simulink model "OrbitSimV1_export"  (R2021b)
settings: Solver=FixedStepAuto  StartTime=0.0  StopTime=1000  FixedStep=.01  RelTol=1e-3
model workspace (MAT data in the model file):
  orbit_altitude = 450000
  r_earth = 6378100
  vel_init = 7640
libraries: matrix_library x5, vrlib x4
settings Model: Creator=Ian Lee  LastModifiedBy=Ian Lee

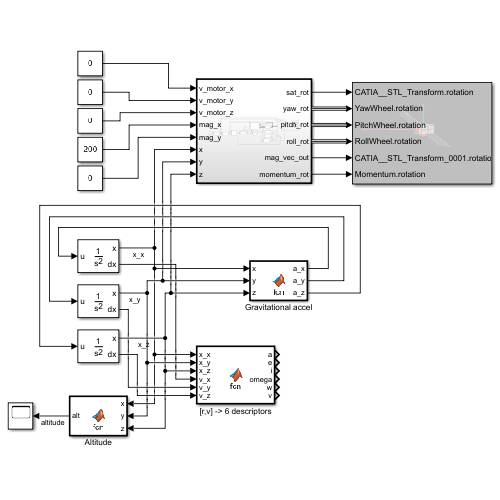
[thumbnail: Simulink's stored preview of the top-level diagram]
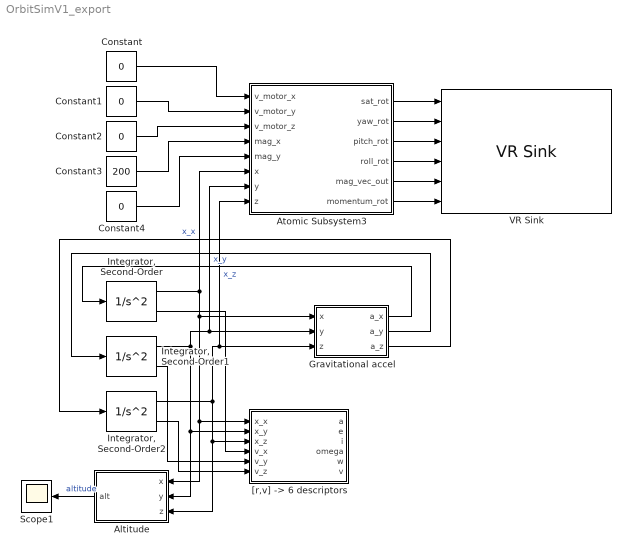
== system OrbitSimV1_export ==
  Altitude : MATLAB Function  TreatAsAtomicUnit=on
  Atomic Subsystem3 : Subsystem  TreatAsAtomicUnit=on
  Constant{,1..2,4} (4 alike) : Constant  Value=0
  Constant3 : Constant  Value=200
  Gravitational accel : MATLAB Function  TreatAsAtomicUnit=on
  "Integrator, Second-Order" : SecondOrderIntegrator  ICX=0  ICDXDT=5500
  "Integrator, Second-Order1" : SecondOrderIntegrator  ICX=r_earth + orbit_altitude  ICDXDT=0
  "Integrator, Second-Order2" : SecondOrderIntegrator  ICDXDT=5300
  Scope1 : Scope
  VR Sink : vrlib/VR Sink  InstantiateOnLoad=on  SampleTime=.02  ViewEnable=on  RemoteChange=off  RemoteView=off  FieldsWritten=CATIA__STL_Transform.rotation.4.1.1.double#YawWheel.rotation.4.1.1.double#PitchWheel.rotation.4.1.1.double#RollWheel.rotation.4.1.1.double#CATIA__STL_Transform_0001.rotation.4.1.1.double#Momentum.rotation.4.1.1.double  WorldFileName=SatVR.x3d  AutoView=off  VideoDimensions=[]  AllowVariableSize=off
  "[r,v] -> 6 descriptors" : MATLAB Function  TreatAsAtomicUnit=on
  wires:
  Gravitational accel/2(a_y) -> "Integrator, Second-Order1"/1
  Gravitational accel/1(a_x) -> "Integrator, Second-Order"/1
  Altitude/1(alt) -> Scope1/1  "altitude"
  "Integrator, Second-Order1"/1 -> "[r,v] -> 6 descriptors"/2(x_y), Altitude/2(y), Atomic Subsystem3/7(y), Gravitational accel/2(y)  "x_y"
  Gravitational accel/3(a_z) -> "Integrator, Second-Order2"/1
  "Integrator, Second-Order2"/1 -> "[r,v] -> 6 descriptors"/3(x_z), Altitude/3(z), Atomic Subsystem3/8(z), Gravitational accel/3(z)  "x_z"
  "Integrator, Second-Order"/1 -> Atomic Subsystem3/6(x), "[r,v] -> 6 descriptors"/1(x_x), Altitude/1(x), Gravitational accel/1(x)  "x_x"
  "Integrator, Second-Order"/2 -> "[r,v] -> 6 descriptors"/4(v_x)
  "Integrator, Second-Order1"/2 -> "[r,v] -> 6 descriptors"/5(v_y)
  "Integrator, Second-Order2"/2 -> "[r,v] -> 6 descriptors"/6(v_z)
  Atomic Subsystem3/1(sat_rot) -> VR Sink/1
  Atomic Subsystem3/2(yaw_rot) -> VR Sink/2
  Atomic Subsystem3/3(pitch_rot) -> VR Sink/3
  Atomic Subsystem3/4(roll_rot) -> VR Sink/4
  Atomic Subsystem3/5(mag_vec_out) -> VR Sink/5
  Atomic Subsystem3/6(momentum_rot) -> VR Sink/6
  Constant4/1 -> Atomic Subsystem3/5(mag_y)
  Constant3/1 -> Atomic Subsystem3/4(mag_x)
  Constant2/1 -> Atomic Subsystem3/3(v_motor_z)
  Constant1/1 -> Atomic Subsystem3/2(v_motor_y)
  Constant/1 -> Atomic Subsystem3/1(v_motor_x)

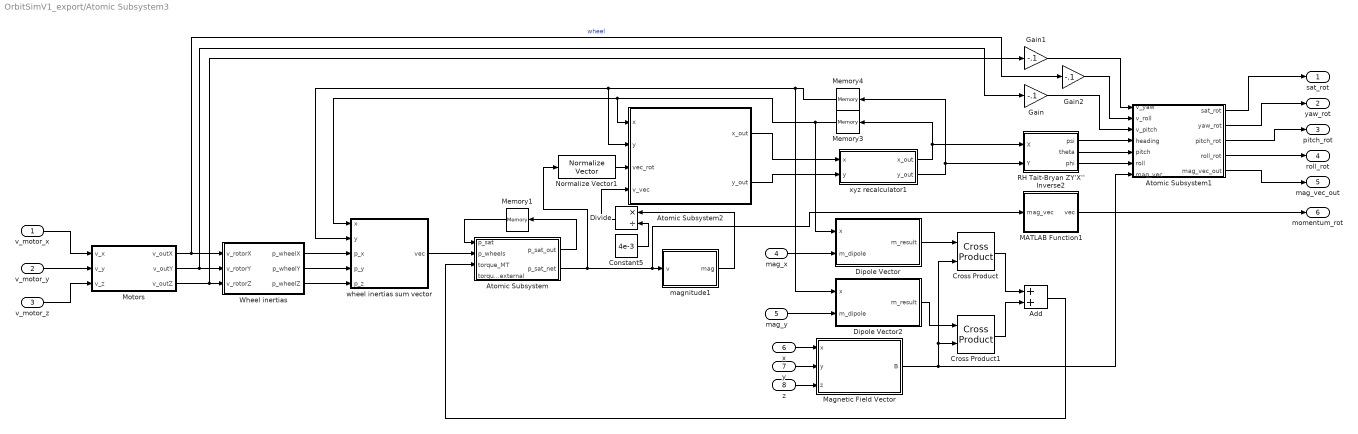
== system OrbitSimV1_export/Atomic Subsystem3 ==
  v_motor_x : Inport
  v_motor_y : Inport  Port=2
  v_motor_z : Inport  Port=3
  mag_x : Inport  Port=4
  mag_y : Inport  Port=5
  x : Inport  Port=6
  y : Inport  Port=7
  z : Inport  Port=8
  Add : Sum
  Atomic Subsystem : Subsystem  TreatAsAtomicUnit=on
  Atomic Subsystem1 : Subsystem  TreatAsAtomicUnit=on
  Atomic Subsystem2 : Subsystem  TreatAsAtomicUnit=on
      mask Display: image('C:\Users\benml\Downloads\imageMas.png'); % Use "Edit Image" on toolstrip to change.
  Constant5 : Constant  Value=4e-3
  Cross Product : matrix_library/Cross Product
      settings: SourceProductBaseCode=SL
  Cross Product1 : matrix_library/Cross Product
      settings: SourceProductBaseCode=SL
  Dipole Vector : MATLAB Function  TreatAsAtomicUnit=on
  Dipole Vector2 : MATLAB Function  TreatAsAtomicUnit=on
  Divide : Product  Inputs=*/
  Gain : Gain  Gain=-.1
  Gain1 : Gain  Gain=-.1
  Gain2 : Gain  Gain=-.1
  MATLAB Function1 : MATLAB Function  TreatAsAtomicUnit=on
  Magnetic Field Vector : MATLAB Function  TreatAsAtomicUnit=on
  Memory1 : Memory
  Memory3 : Memory  InitialCondition=[1,0,0]
  Memory4 : Memory  InitialCondition=[0,1,0]
  Motors : Subsystem  TreatAsAtomicUnit=on
  Normalize Vector1 : vrlib/Utilities/Normalize Vector  maxzero=0
  RH Tait-Bryan ZY'X'' Inverse2 : MATLAB Function  TreatAsAtomicUnit=on
  Wheel inertias : Subsystem  TreatAsAtomicUnit=on
  magnitude1 : MATLAB Function  TreatAsAtomicUnit=on
  wheel inertias sum vector : Subsystem  TreatAsAtomicUnit=on
  xyz recalculator1 : Subsystem  TreatAsAtomicUnit=on
  sat_rot : Outport
  yaw_rot : Outport  Port=2
  pitch_rot : Outport  Port=3
  roll_rot : Outport  Port=4
  mag_vec_out : Outport  Port=5
  momentum_rot : Outport  Port=6
  wires:
  wheel inertias sum vector/1(" vec") -> Atomic Subsystem/2(p_wheels)
  Atomic Subsystem/2(p_sat_net) -> MATLAB Function1/1(mag_vec), magnitude1/1(v), Normalize Vector1/1
  Normalize Vector1/1 -> Atomic Subsystem2/3(vec_rot)
  Memory1/1 -> Atomic Subsystem/1(p_sat)
  Atomic Subsystem/1(p_sat_out) -> Memory1/1
  Cross Product1/1 -> Add/2
  Add/1 -> Atomic Subsystem/3(torque_MT)
  Constant5/1 -> Divide/2
  Divide/1 -> Atomic Subsystem2/4(v_vec)
  xyz recalculator1/1(x_out) -> RH Tait-Bryan ZY'X'' Inverse2/1(X), Memory3/1
  RH Tait-Bryan ZY'X'' Inverse2/2(theta) -> Atomic Subsystem1/5(pitch)
  RH Tait-Bryan ZY'X'' Inverse2/1(psi) -> Atomic Subsystem1/4(heading)
  Atomic Subsystem2/1(x_out) -> xyz recalculator1/1(x)
  Cross Product/1 -> Add/1
  Gain/1 -> Atomic Subsystem1/3(v_pitch)
  MATLAB Function1/1(vec) -> momentum_rot/1
  Atomic Subsystem2/2(y_out) -> xyz recalculator1/2(y)
  Magnetic Field Vector/1(B) -> Cross Product/2, Cross Product1/2, Atomic Subsystem1/7(mag_vec)
  Gain2/1 -> Atomic Subsystem1/2(v_roll)
  Atomic Subsystem1/2(yaw_rot) -> yaw_rot/1
  Wheel inertias/3(p_wheelZ) -> wheel inertias sum vector/5(p_z)
  Atomic Subsystem1/3(pitch_rot) -> pitch_rot/1
  Motors/1(v_outX) -> Gain2/1, Wheel inertias/1(v_rotorX)  "wheel"
  xyz recalculator1/2(y_out) -> RH Tait-Bryan ZY'X'' Inverse2/2(Y), Memory4/1
  RH Tait-Bryan ZY'X'' Inverse2/3(phi) -> Atomic Subsystem1/6(roll)
  Motors/3(v_outZ) -> Gain1/1, Wheel inertias/3(v_rotorZ)
  Motors/2(v_outY) -> Gain/1, Wheel inertias/2(v_rotorY)
  Wheel inertias/2(p_wheelY) -> wheel inertias sum vector/4(p_y)
  Atomic Subsystem1/1(sat_rot) -> sat_rot/1
  Gain1/1 -> Atomic Subsystem1/1(v_yaw)
  Dipole Vector/1(m_result) -> Cross Product/1
  Memory3/1 -> Dipole Vector/1(x), wheel inertias sum vector/1(x), Atomic Subsystem2/1(x)
  Dipole Vector2/1(m_result) -> Cross Product1/1
  Atomic Subsystem1/5(mag_vec_out) -> mag_vec_out/1
  magnitude1/1(mag) -> Divide/1
  Memory4/1 -> Atomic Subsystem2/2(y), wheel inertias sum vector/2(y), Dipole Vector2/1(x)
  Wheel inertias/1(p_wheelX) -> wheel inertias sum vector/3(p_x)
  Atomic Subsystem1/4(roll_rot) -> roll_rot/1
  z/1 -> Magnetic Field Vector/3(z)
  y/1 -> Magnetic Field Vector/2(y)
  x/1 -> Magnetic Field Vector/1(x)
  v_motor_y/1 -> Motors/2(v_y)
  v_motor_x/1 -> Motors/1(v_x)
  v_motor_z/1 -> Motors/3(v_z)
  mag_x/1 -> Dipole Vector/2(m_dipole)
  mag_y/1 -> Dipole Vector2/2(m_dipole)

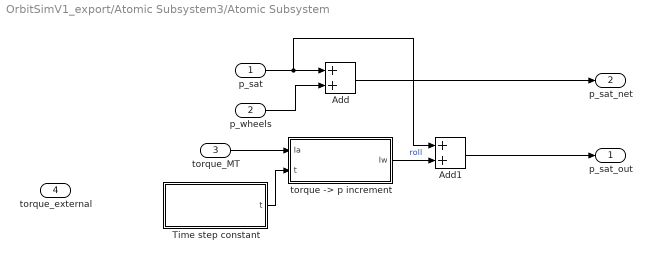
== system OrbitSimV1_export/Atomic Subsystem3/Atomic Subsystem ==
  p_sat : Inport
  p_wheels : Inport  Port=2
  torque_MT : Inport  Port=3
  torque_external : Inport  Port=4
  Add : Sum
  Add1 : Sum
  Time step constant : Subsystem  TreatAsAtomicUnit=on
  "torque -> p increment" : Subsystem  TreatAsAtomicUnit=on
  p_sat_out : Outport
  p_sat_net : Outport  Port=2
  wires:
  Time step constant/1(t) -> "torque -> p increment"/2(t)
  torque_MT/1 -> "torque -> p increment"/1(Ia)
  p_sat/1 -> Add1/1, Add/1
  p_wheels/1 -> Add/2
  Add/1 -> p_sat_net/1
  "torque -> p increment"/1(Iw) -> Add1/2  "roll"
  Add1/1 -> p_sat_out/1

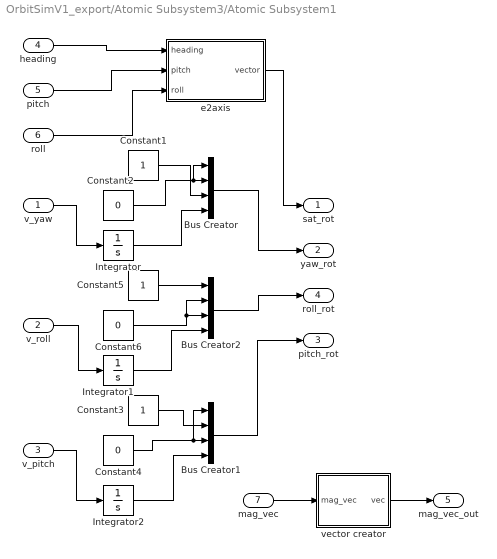
== system OrbitSimV1_export/Atomic Subsystem3/Atomic Subsystem1 ==
  v_yaw : Inport
  v_roll : Inport  Port=2
  v_pitch : Inport  Port=3
  heading : Inport  Port=4
  pitch : Inport  Port=5
  roll : Inport  Port=6
  mag_vec : Inport  Port=7
  Bus Creator : BusCreator  Inputs=4
  Bus Creator1 : BusCreator  Inputs=4
  Bus Creator2 : BusCreator  Inputs=4
  Constant1 : Constant
  Constant2 : Constant  Value=0
  Constant3 : Constant
  Constant4 : Constant  Value=0
  Constant5 : Constant
  Constant6 : Constant  Value=0
  Integrator : Integrator
  Integrator1 : Integrator
  Integrator2 : Integrator
  e2axis : MATLAB Function  TreatAsAtomicUnit=on
  vector creator : MATLAB Function  TreatAsAtomicUnit=on
  sat_rot : Outport
  yaw_rot : Outport  Port=2
  pitch_rot : Outport  Port=3
  roll_rot : Outport  Port=4
  mag_vec_out : Outport  Port=5
  wires:
  Constant6/1 -> Bus Creator2/2, Bus Creator2/3
  Constant5/1 -> Bus Creator2/1
  Constant1/1 -> Bus Creator/3
  Constant3/1 -> Bus Creator1/2
  Constant2/1 -> Bus Creator/1, Bus Creator/2
  Constant4/1 -> Bus Creator1/1, Bus Creator1/3
  heading/1 -> e2axis/1(heading)
  pitch/1 -> e2axis/2(pitch)
  roll/1 -> e2axis/3(roll)
  e2axis/1(vector) -> sat_rot/1
  v_yaw/1 -> Integrator/1
  v_roll/1 -> Integrator1/1
  v_pitch/1 -> Integrator2/1
  Bus Creator/1 -> yaw_rot/1
  Bus Creator2/1 -> roll_rot/1
  Bus Creator1/1 -> pitch_rot/1
  Integrator/1 -> Bus Creator/4
  Integrator1/1 -> Bus Creator2/4
  Integrator2/1 -> Bus Creator1/4
  mag_vec/1 -> vector creator/1(mag_vec)
  vector creator/1(vec) -> mag_vec_out/1

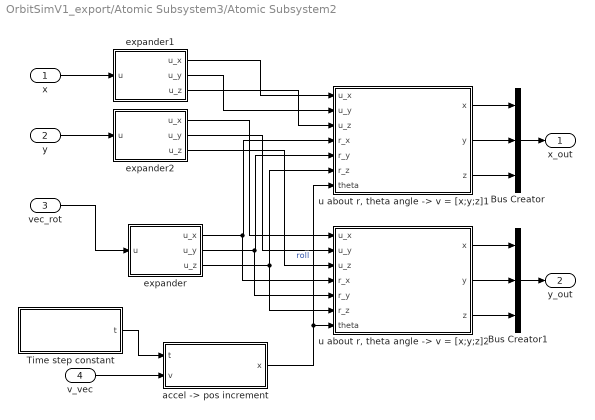
== system OrbitSimV1_export/Atomic Subsystem3/Atomic Subsystem2 ==
  x : Inport
  y : Inport  Port=2
  vec_rot : Inport  Port=3
  v_vec : Inport  Port=4
  Bus Creator : BusCreator  Inputs=3
  Bus Creator1 : BusCreator  Inputs=3
  Time step constant : Subsystem  TreatAsAtomicUnit=on
  "accel -> pos increment" : Subsystem  TreatAsAtomicUnit=on
  expander : MATLAB Function  TreatAsAtomicUnit=on
  expander1 : MATLAB Function  TreatAsAtomicUnit=on
  expander2 : MATLAB Function  TreatAsAtomicUnit=on
  "u about r, theta angle -> v = [x;y;z]1" : Subsystem  TreatAsAtomicUnit=on
  "u about r, theta angle -> v = [x;y;z]2" : Subsystem  TreatAsAtomicUnit=on
  x_out : Outport
  y_out : Outport  Port=2
  wires:
  x/1 -> expander1/1(u)
  vec_rot/1 -> expander/1(u)
  expander1/1(u_x) -> "u about r, theta angle -> v = [x;y;z]1"/1(u_x)
  expander1/2(u_y) -> "u about r, theta angle -> v = [x;y;z]1"/2(u_y)
  expander1/3(u_z) -> "u about r, theta angle -> v = [x;y;z]1"/3(u_z)
  expander/1(u_x) -> "u about r, theta angle -> v = [x;y;z]2"/4(r_x), "u about r, theta angle -> v = [x;y;z]1"/4(r_x)
  expander/2(u_y) -> "u about r, theta angle -> v = [x;y;z]2"/5(r_y), "u about r, theta angle -> v = [x;y;z]1"/5(r_y)
  expander/3(u_z) -> "u about r, theta angle -> v = [x;y;z]1"/6(r_z), "u about r, theta angle -> v = [x;y;z]2"/6(r_z)
  expander2/1(u_x) -> "u about r, theta angle -> v = [x;y;z]2"/1(u_x)
  expander2/2(u_y) -> "u about r, theta angle -> v = [x;y;z]2"/2(u_y)
  expander2/3(u_z) -> "u about r, theta angle -> v = [x;y;z]2"/3(u_z)
  y/1 -> expander2/1(u)
  Time step constant/1(t) -> "accel -> pos increment"/1(t)
  "accel -> pos increment"/1(x) -> "u about r, theta angle -> v = [x;y;z]1"/7(theta), "u about r, theta angle -> v = [x;y;z]2"/7(theta)  "roll"
  v_vec/1 -> "accel -> pos increment"/2("v ")
  "u about r, theta angle -> v = [x;y;z]1"/1(x) -> Bus Creator/1
  "u about r, theta angle -> v = [x;y;z]1"/2(y) -> Bus Creator/2
  "u about r, theta angle -> v = [x;y;z]1"/3(z) -> Bus Creator/3
  Bus Creator/1 -> x_out/1
  Bus Creator1/1 -> y_out/1
  "u about r, theta angle -> v = [x;y;z]2"/2(y) -> Bus Creator1/2
  "u about r, theta angle -> v = [x;y;z]2"/1(x) -> Bus Creator1/1
  "u about r, theta angle -> v = [x;y;z]2"/3(z) -> Bus Creator1/3

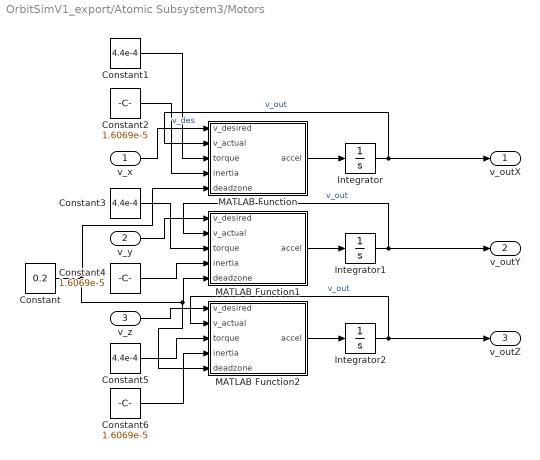
== system OrbitSimV1_export/Atomic Subsystem3/Motors ==
  v_x : Inport
  v_y : Inport  Port=2
  v_z : Inport  Port=3
  Constant : Constant  Value=0.2
  Constant1 : Constant  Value=4.4e-4
  Constant2 : Constant  Value=1.6069e-5
  Constant3 : Constant  Value=4.4e-4
  Constant4 : Constant  Value=1.6069e-5
  Constant5 : Constant  Value=4.4e-4
  Constant6 : Constant  Value=1.6069e-5
  Integrator : Integrator
  Integrator1 : Integrator
  Integrator2 : Integrator
  MATLAB Function : MATLAB Function  TreatAsAtomicUnit=on
  MATLAB Function1 : MATLAB Function  TreatAsAtomicUnit=on
  MATLAB Function2 : MATLAB Function  TreatAsAtomicUnit=on
  v_outX : Outport
  v_outY : Outport  Port=2
  v_outZ : Outport  Port=3
  wires:
  Constant1/1 -> MATLAB Function/3(torque)
  Constant2/1 -> MATLAB Function/4(inertia)
  MATLAB Function/1(accel) -> Integrator/1
  Integrator/1 -> MATLAB Function/2(v_actual), v_outX/1  "v_out"
  v_x/1 -> MATLAB Function/1(v_desired)  "v_des"
  Constant3/1 -> MATLAB Function1/3(torque)
  Constant4/1 -> MATLAB Function1/4(inertia)
  MATLAB Function1/1(accel) -> Integrator1/1
  Integrator1/1 -> v_outY/1, MATLAB Function1/2(v_actual)  "v_out"
  v_y/1 -> MATLAB Function1/1(v_desired)
  Constant5/1 -> MATLAB Function2/3(torque)
  Constant6/1 -> MATLAB Function2/4(inertia)
  MATLAB Function2/1(accel) -> Integrator2/1
  Integrator2/1 -> MATLAB Function2/2(v_actual), v_outZ/1  "v_out"
  v_z/1 -> MATLAB Function2/1(v_desired)
  Constant/1 -> MATLAB Function2/5(deadzone), MATLAB Function1/5(deadzone), MATLAB Function/5(deadzone)

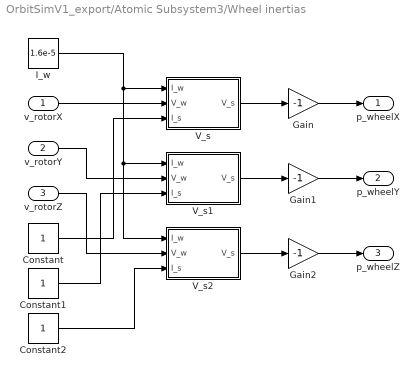
== system OrbitSimV1_export/Atomic Subsystem3/Wheel inertias ==
  v_rotorX : Inport
  v_rotorY : Inport  Port=2
  v_rotorZ : Inport  Port=3
  Constant : Constant
  Constant1 : Constant
  Constant2 : Constant
  Gain : Gain  Gain=-1
  Gain1 : Gain  Gain=-1
  Gain2 : Gain  Gain=-1
  I_w : Constant  Value=1.6e-5
  V_s : MATLAB Function  TreatAsAtomicUnit=on
  V_s1 : MATLAB Function  TreatAsAtomicUnit=on
  V_s2 : MATLAB Function  TreatAsAtomicUnit=on
  p_wheelX : Outport
  p_wheelY : Outport  Port=2
  p_wheelZ : Outport  Port=3
  wires:
  I_w/1 -> V_s2/1(I_w), V_s1/1(I_w), V_s/1(I_w)
  v_rotorX/1 -> V_s/2(V_w)
  Constant/1 -> V_s/3(I_s)
  v_rotorY/1 -> V_s1/2(V_w)
  v_rotorZ/1 -> V_s2/2(V_w)
  Constant1/1 -> V_s1/3(I_s)
  Constant2/1 -> V_s2/3(I_s)
  V_s/1(V_s) -> Gain/1
  V_s1/1(V_s) -> Gain1/1
  V_s2/1(V_s) -> Gain2/1
  Gain2/1 -> p_wheelZ/1
  Gain1/1 -> p_wheelY/1
  Gain/1 -> p_wheelX/1

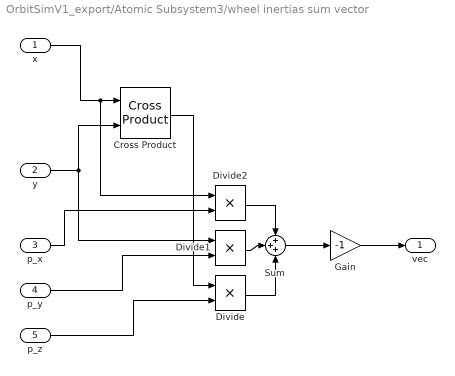
== system OrbitSimV1_export/Atomic Subsystem3/wheel inertias sum vector ==
  x : Inport
  y : Inport  Port=2
  p_x : Inport  Port=3
  p_y : Inport  Port=4
  p_z : Inport  Port=5
  Cross Product : matrix_library/Cross Product
      settings: SourceProductBaseCode=SL
  Divide : Product  Inputs=**
  Divide1 : Product  Inputs=**
  Divide2 : Product  Inputs=**
  Gain : Gain  Gain=-1
  Sum : Sum  Inputs=+++
  " vec" : Outport
  wires:
  x/1 -> Divide2/1, Cross Product/1
  y/1 -> Divide1/1, Cross Product/2
  Cross Product/1 -> Divide/1
  p_z/1 -> Divide/2
  p_x/1 -> Divide2/2
  p_y/1 -> Divide1/2
  Divide1/1 -> Sum/2
  Divide2/1 -> Sum/1
  Divide/1 -> Sum/3
  Gain/1 -> " vec"/1
  Sum/1 -> Gain/1

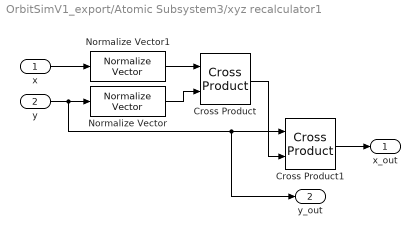
== system OrbitSimV1_export/Atomic Subsystem3/xyz recalculator1 ==
  x : Inport
  y : Inport  Port=2
  Cross Product : matrix_library/Cross Product
      settings: SourceProductBaseCode=SL
  Cross Product1 : matrix_library/Cross Product
      settings: SourceProductBaseCode=SL
  Normalize Vector : vrlib/Utilities/Normalize Vector  maxzero=0
  Normalize Vector1 : vrlib/Utilities/Normalize Vector  maxzero=0
  x_out : Outport
  y_out : Outport  Port=2
  wires:
  x/1 -> Normalize Vector1/1
  y/1 -> y_out/1, Cross Product1/1, Normalize Vector/1
  Normalize Vector1/1 -> Cross Product/1
  Normalize Vector/1 -> Cross Product/2
  Cross Product/1 -> Cross Product1/2
  Cross Product1/1 -> x_out/1

== system OrbitSimV1_export/Atomic Subsystem3/Atomic Subsystem/Time step constant ==
  Clock : Clock
  Memory : Memory  InitialCondition=0.1
  Subtract : Sum  Inputs=+-
  t : Outport
  wires:
  Clock/1 -> Memory/1, Subtract/1
  Memory/1 -> Subtract/2
  Subtract/1 -> t/1

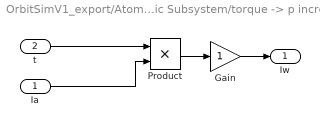
== system OrbitSimV1_export/Atomic Subsystem3/Atomic Subsystem/torque -> p increment ==
  Ia : Inport
  t : Inport  Port=2
  Gain : Gain
  Product : Product
  Iw : Outport
  wires:
  t/1 -> Product/1
  Ia/1 -> Product/2
  Product/1 -> Gain/1
  Gain/1 -> Iw/1

== system OrbitSimV1_export/Atomic Subsystem3/Atomic Subsystem2/Time step constant ==
  Clock : Clock
  Memory : Memory  InitialCondition=0.1
  Subtract : Sum  Inputs=+-
  t : Outport
  wires:
  Clock/1 -> Memory/1, Subtract/1
  Memory/1 -> Subtract/2
  Subtract/1 -> t/1

== system OrbitSimV1_export/Atomic Subsystem3/Atomic Subsystem2/accel -> pos increment ==
  t : Inport
  "v " : Inport  Port=2
  Gain : Gain
  Product : Product
  x : Outport
  wires:
  t/1 -> Product/1
  "v "/1 -> Product/2
  Product/1 -> Gain/1
  Gain/1 -> x/1

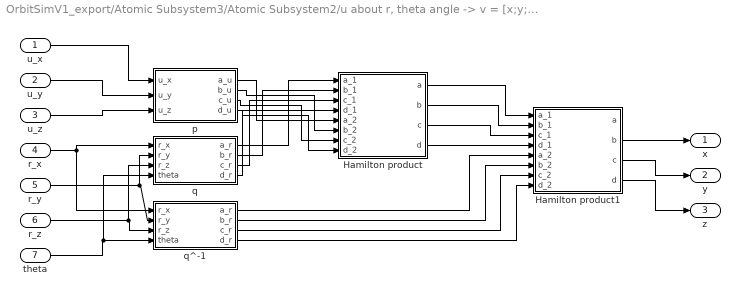
== system OrbitSimV1_export/Atomic Subsystem3/Atomic Subsystem2/u about r, theta angle -> v = [x;y;z]1 ==
  u_x : Inport
  u_y : Inport  Port=2
  u_z : Inport  Port=3
  r_x : Inport  Port=4
  r_y : Inport  Port=5
  r_z : Inport  Port=6
  theta : Inport  Port=7
  Hamilton product : MATLAB Function  TreatAsAtomicUnit=on
  Hamilton product1 : MATLAB Function  TreatAsAtomicUnit=on
  p : MATLAB Function  TreatAsAtomicUnit=on
  q : MATLAB Function  TreatAsAtomicUnit=on
  q^-1 : MATLAB Function  TreatAsAtomicUnit=on
  x : Outport
  y : Outport  Port=2
  z : Outport  Port=3
  wires:
  Hamilton product/1(a) -> Hamilton product1/1(a_1)
  Hamilton product/2(b) -> Hamilton product1/2(b_1)
  Hamilton product/3(c) -> Hamilton product1/3(c_1)
  Hamilton product/4(d) -> Hamilton product1/4(d_1)
  q^-1/1(a_r) -> Hamilton product1/5(a_2)
  q^-1/2(b_r) -> Hamilton product1/6(b_2)
  q^-1/3(c_r) -> Hamilton product1/7(c_2)
  q^-1/4(d_r) -> Hamilton product1/8(d_2)
  theta/1 -> q/4(theta), q^-1/4(theta)
  r_z/1 -> q/3(r_z), q^-1/3(r_z)
  r_y/1 -> q/2(r_y), q^-1/2(r_y)
  r_x/1 -> q/1(r_x), q^-1/1(r_x)
  u_z/1 -> p/3(u_z)
  u_y/1 -> p/2(u_y)
  u_x/1 -> p/1(u_x)
  Hamilton product1/2(b) -> x/1
  Hamilton product1/3(c) -> y/1
  Hamilton product1/4(d) -> z/1
  q/1(a_r) -> Hamilton product/1(a_1)
  q/2(b_r) -> Hamilton product/2(b_1)
  q/3(c_r) -> Hamilton product/3(c_1)
  q/4(d_r) -> Hamilton product/4(d_1)
  p/2(b_u) -> Hamilton product/6(b_2)
  p/3(c_u) -> Hamilton product/7(c_2)
  p/4(d_u) -> Hamilton product/8(d_2)
  p/1(a_u) -> Hamilton product/5(a_2)

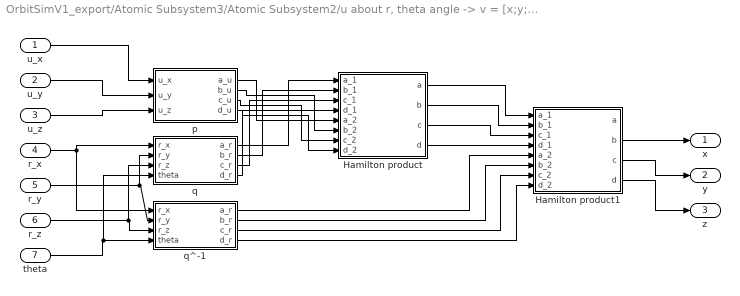
== system OrbitSimV1_export/Atomic Subsystem3/Atomic Subsystem2/u about r, theta angle -> v = [x;y;z]2 ==
  u_x : Inport
  u_y : Inport  Port=2
  u_z : Inport  Port=3
  r_x : Inport  Port=4
  r_y : Inport  Port=5
  r_z : Inport  Port=6
  theta : Inport  Port=7
  Hamilton product : MATLAB Function  TreatAsAtomicUnit=on
  Hamilton product1 : MATLAB Function  TreatAsAtomicUnit=on
  p : MATLAB Function  TreatAsAtomicUnit=on
  q : MATLAB Function  TreatAsAtomicUnit=on
  q^-1 : MATLAB Function  TreatAsAtomicUnit=on
  x : Outport
  y : Outport  Port=2
  z : Outport  Port=3
  wires:
  Hamilton product/1(a) -> Hamilton product1/1(a_1)
  Hamilton product/2(b) -> Hamilton product1/2(b_1)
  Hamilton product/3(c) -> Hamilton product1/3(c_1)
  Hamilton product/4(d) -> Hamilton product1/4(d_1)
  q^-1/1(a_r) -> Hamilton product1/5(a_2)
  q^-1/2(b_r) -> Hamilton product1/6(b_2)
  q^-1/3(c_r) -> Hamilton product1/7(c_2)
  q^-1/4(d_r) -> Hamilton product1/8(d_2)
  theta/1 -> q/4(theta), q^-1/4(theta)
  r_z/1 -> q/3(r_z), q^-1/3(r_z)
  r_y/1 -> q/2(r_y), q^-1/2(r_y)
  r_x/1 -> q/1(r_x), q^-1/1(r_x)
  u_z/1 -> p/3(u_z)
  u_y/1 -> p/2(u_y)
  u_x/1 -> p/1(u_x)
  Hamilton product1/2(b) -> x/1
  Hamilton product1/3(c) -> y/1
  Hamilton product1/4(d) -> z/1
  q/1(a_r) -> Hamilton product/1(a_1)
  q/2(b_r) -> Hamilton product/2(b_1)
  q/3(c_r) -> Hamilton product/3(c_1)
  q/4(d_r) -> Hamilton product/4(d_1)
  p/2(b_u) -> Hamilton product/6(b_2)
  p/3(c_u) -> Hamilton product/7(c_2)
  p/4(d_u) -> Hamilton product/8(d_2)
  p/1(a_u) -> Hamilton product/5(a_2)

== matlab function OrbitSimV1_export/Atomic Subsystem3/Atomic Subsystem2/u about r, theta angle -> v = [x;y;z]1/Hamilton product ==
  data: a_1 input; a output; b_1 input; c_1 input; d_1 input; a_2 input; b_2 input; c_2 input; d_2 input; b output; c output; d output
function [a, b, c, d] = fcn(a_1, b_1, c_1, d_1, a_2, b_2, c_2, d_2)

a = a_1 * a_2 - b_1 * b_2 - c_1 * c_2 - d_1 * d_2;
b = a_1 * b_2 + b_1 * a_2 + c_1 * d_2 - d_1 * c_2;
c = a_1 * c_2 - b_1 * d_2 + c_1 * a_2 + d_1 * b_2;
d = a_1 * d_2 + b_1 * c_2 - c_1 * b_2 + d_1 * a_2;

== matlab function OrbitSimV1_export/Atomic Subsystem3/Atomic Subsystem2/u about r, theta angle -> v = [x;y;z]1/Hamilton product1 ==
  data: a_1 input; a output; b_1 input; c_1 input; d_1 input; a_2 input; b_2 input; c_2 input; d_2 input; b output; c output; d output
function [a, b, c, d] = fcn(a_1, b_1, c_1, d_1, a_2, b_2, c_2, d_2)

a = a_1 * a_2 - b_1 * b_2 - c_1 * c_2 - d_1 * d_2;
b = a_1 * b_2 + b_1 * a_2 + c_1 * d_2 - d_1 * c_2;
c = a_1 * c_2 - b_1 * d_2 + c_1 * a_2 + d_1 * b_2;
d = a_1 * d_2 + b_1 * c_2 - c_1 * b_2 + d_1 * a_2;

== matlab function OrbitSimV1_export/Atomic Subsystem3/Atomic Subsystem2/u about r, theta angle -> v = [x;y;z]1/p ==
  data: u_x input; u_y input; u_z input; a_u output; b_u output; c_u output; d_u output
function [a_u, b_u, c_u, d_u] = fcn(u_x, u_y, u_z)
a_u = 0;
b_u = u_x;
c_u = u_y;
d_u = u_z;

== matlab function OrbitSimV1_export/Atomic Subsystem3/Atomic Subsystem2/u about r, theta angle -> v = [x;y;z]1/q ==
  data: r_x input; a_r output; r_y input; r_z input; theta input; b_r output; c_r output; d_r output
function [a_r, b_r, c_r, d_r] = fcn(r_x, r_y, r_z, theta)

a_r = cos(theta / 2);
b_r = r_x * sin(theta / 2);
c_r = r_y * sin(theta / 2);
d_r = r_z * sin(theta / 2);

== matlab function OrbitSimV1_export/Atomic Subsystem3/Atomic Subsystem2/u about r, theta angle -> v = [x;y;z]1/q^-1 ==
  data: r_x input; a_r output; r_y input; r_z input; theta input; b_r output; c_r output; d_r output
function [a_r, b_r, c_r, d_r] = fcn(r_x, r_y, r_z, theta)

a_r = cos(theta / 2);
b_r = r_x * -sin(theta / 2);
c_r = r_y * -sin(theta / 2);
d_r = r_z * -sin(theta / 2);

== matlab function OrbitSimV1_export/Atomic Subsystem3/Atomic Subsystem2/u about r, theta angle -> v = [x;y;z]2/Hamilton product ==
  data: a_1 input; a output; b_1 input; c_1 input; d_1 input; a_2 input; b_2 input; c_2 input; d_2 input; b output; c output; d output
function [a, b, c, d] = fcn(a_1, b_1, c_1, d_1, a_2, b_2, c_2, d_2)

a = a_1 * a_2 - b_1 * b_2 - c_1 * c_2 - d_1 * d_2;
b = a_1 * b_2 + b_1 * a_2 + c_1 * d_2 - d_1 * c_2;
c = a_1 * c_2 - b_1 * d_2 + c_1 * a_2 + d_1 * b_2;
d = a_1 * d_2 + b_1 * c_2 - c_1 * b_2 + d_1 * a_2;

== matlab function OrbitSimV1_export/Atomic Subsystem3/Atomic Subsystem2/u about r, theta angle -> v = [x;y;z]2/Hamilton product1 ==
  data: a_1 input; a output; b_1 input; c_1 input; d_1 input; a_2 input; b_2 input; c_2 input; d_2 input; b output; c output; d output
function [a, b, c, d] = fcn(a_1, b_1, c_1, d_1, a_2, b_2, c_2, d_2)

a = a_1 * a_2 - b_1 * b_2 - c_1 * c_2 - d_1 * d_2;
b = a_1 * b_2 + b_1 * a_2 + c_1 * d_2 - d_1 * c_2;
c = a_1 * c_2 - b_1 * d_2 + c_1 * a_2 + d_1 * b_2;
d = a_1 * d_2 + b_1 * c_2 - c_1 * b_2 + d_1 * a_2;

== matlab function OrbitSimV1_export/Atomic Subsystem3/Atomic Subsystem2/u about r, theta angle -> v = [x;y;z]2/p ==
  data: u_x input; u_y input; u_z input; a_u output; b_u output; c_u output; d_u output
function [a_u, b_u, c_u, d_u] = fcn(u_x, u_y, u_z)
a_u = 0;
b_u = u_x;
c_u = u_y;
d_u = u_z;

== matlab function OrbitSimV1_export/Gravitational accel ==
  data: x input; a_x output; y input; z input; a_y output; a_z output
function [a_x, a_y, a_z] = fcn(x, y, z)
% determine acceleration
d = sqrt(x^2 + y^2 + z^2);
a = -((6.67408*10^-11) * (5.97219*10^24)) / d^2;
% x,y,z unit vector for direction
x1 = x / d;
y1 = y / d;
z1 = z / d;
% x,y,z acceleration vectors
a_x = a * x1;
a_y = a * y1;
a_z = a * z1;

== matlab function OrbitSimV1_export/Atomic Subsystem3/Atomic Subsystem2/u about r, theta angle -> v = [x;y;z]2/q ==
  data: r_x input; a_r output; r_y input; r_z input; theta input; b_r output; c_r output; d_r output
function [a_r, b_r, c_r, d_r] = fcn(r_x, r_y, r_z, theta)

a_r = cos(theta / 2);
b_r = r_x * sin(theta / 2);
c_r = r_y * sin(theta / 2);
d_r = r_z * sin(theta / 2);

== matlab function OrbitSimV1_export/Atomic Subsystem3/Atomic Subsystem2/u about r, theta angle -> v = [x;y;z]2/q^-1 ==
  data: r_x input; a_r output; r_y input; r_z input; theta input; b_r output; c_r output; d_r output
function [a_r, b_r, c_r, d_r] = fcn(r_x, r_y, r_z, theta)

a_r = cos(theta / 2);
b_r = r_x * -sin(theta / 2);
c_r = r_y * -sin(theta / 2);
d_r = r_z * -sin(theta / 2);

== matlab function OrbitSimV1_export/Atomic Subsystem3/Dipole Vector ==
  data: x input; m_result output; m_dipole input
function m_result  = fcn(x,m_dipole)

m_result = [0;0;0];
mag = sqrt(x(1)^2 + x(2)^2 + x(3)^2);
m_result(1) = m_dipole * (x(1) / mag);
m_result(2) = m_dipole * (x(2) / mag);
m_result(3) = m_dipole * (x(3) / mag);

== matlab function OrbitSimV1_export/Atomic Subsystem3/Dipole Vector2 ==
  data: x input; m_result output; m_dipole input
function m_result  = fcn(x,m_dipole)

m_result = [0;0;0];
mag = sqrt(x(1)^2 + x(2)^2 + x(3)^2);
m_result(1) = m_dipole * (x(1) / mag);
m_result(2) = m_dipole * (x(2) / mag);
m_result(3) = m_dipole * (x(3) / mag);

== matlab function OrbitSimV1_export/Atomic Subsystem3/MATLAB Function1 ==
  data: mag_vec input; vec output
function vec = fcn(mag_vec)

cos_theta = mag_vec(3) / sqrt(mag_vec(1)^2+mag_vec(2)^2+mag_vec(3)^2);
theta = acos(cos_theta);
vec = [-mag_vec(2); mag_vec(1); 0; theta];

== matlab function OrbitSimV1_export/Atomic Subsystem3/Magnetic Field Vector ==
  data: x input; B output; y input; z input
function B  = fcn(x,y,z)

B = [0;0;0];
q1 = 150; % bottom charge
q2 = 180; % top charge
r_earth = 6.3781e6;
inset = 2/3;
d_t = x^2 + y^2 + (z - r_earth * inset)^2; % distance squared from top charge to point
d_b = x^2 + y^2 + (z + r_earth * inset)^2; % distance squared from bottom charge to point

B(1) = (x) * (q1 / d_b - q2 / d_t);
B(2) = (y) * (q1 / d_b - q2 / d_t);
B(3) = (q1 / d_b) * (z + r_earth * inset) - (q1 / d_t) * (z - r_earth * inset);

== matlab function OrbitSimV1_export/Atomic Subsystem3/Motors/MATLAB Function ==
  data: v_desired input; accel output; v_actual input; torque input; inertia input; deadzone input
function accel  = fcn(v_desired, v_actual, torque, inertia, deadzone)
if(v_desired - deadzone > v_actual)
    accel = torque / inertia;
elseif(v_desired + deadzone < v_actual)
    accel = -torque / inertia;
else
    accel = 0;
end

== matlab function OrbitSimV1_export/Atomic Subsystem3/Motors/MATLAB Function1 ==
  data: v_desired input; accel output; v_actual input; torque input; inertia input; deadzone input
function accel  = fcn(v_desired, v_actual, torque, inertia, deadzone)
if(v_desired - deadzone > v_actual)
    accel = torque / inertia;
elseif(v_desired + deadzone < v_actual)
    accel = -torque / inertia;
else
    accel = 0;
end

== matlab function OrbitSimV1_export/Atomic Subsystem3/Motors/MATLAB Function2 ==
  data: v_desired input; accel output; v_actual input; torque input; inertia input; deadzone input
function accel  = fcn(v_desired, v_actual, torque, inertia, deadzone)
if(v_desired - deadzone > v_actual)
    accel = torque / inertia;
elseif(v_desired + deadzone < v_actual)
    accel = -torque / inertia;
else
    accel = 0;
end

== matlab function OrbitSimV1_export/Atomic Subsystem3/RH Tait-Bryan ZY'X'' Inverse2 ==
  data: X input; psi output; Y input; theta output; phi output
function [psi, theta, phi] = fcn(X,Y)

% psi = heading
% theta = pitch
% phi = bank

psi = atan2(X(2),X(1));
theta = atan2(X(3),sqrt(X(2)^2 + X(1)^2));
if(-Y(1) * sin(psi) + Y(2) * cos(psi) > 1)
    n = 1;
elseif(-Y(1) * sin(psi) + Y(2) * cos(psi) < -1)
    n = -1;
else
    n = -Y(1) * sin(psi) + Y(2) * cos(psi);
end
if(Y(3) > 0)
    phi = acos(n);
else
    phi = -acos(n);
end

== matlab function OrbitSimV1_export/Atomic Subsystem3/Wheel inertias/V_s ==
  data: I_w input; V_s output; V_w input; I_s input
function V_s = fcn(I_w, V_w, I_s)
V_s = (I_w * V_w) / I_s;

== matlab function OrbitSimV1_export/[r,v] -> 6 descriptors ==
  data: x_x input; a output; x_y input; x_z input; v_x input; v_y input; v_z input; e output; i output; omega output; w output; v output
function [a, e, i, omega, w, v] = fcn(x_x, x_y, x_z, v_x, v_y, v_z)

% by math magic, we know (SEE RESEARCH FILES\Orbital mechanics.pdf):
% e is the eccentricity vector, that points from apoapsis to periapsis with
% magnitude = orbit's scalar eccentricity; mu is standard gravitational
% parameter: mu = G(m1 + m2), in this case satellite mass is negligible. 

r = [x_x, x_y, x_z];
r_hat = r / norm(r);
r_dot = [v_x, v_y, v_z];
h = cross(r,r_dot);
mu = 3.986004418*10^14;
ecc_vec = (1 / mu) * (cross(r_dot,h) - mu * r_hat);
e = norm(ecc_vec); % e

i = acos(h(3) / norm(h)); % i

spec_mech_e = ((norm(r_dot))^2 / 2) - mu / norm(r);
a = (-mu) / (2 * spec_mech_e); % a

if(i ~= 0)
    n = cross([0,0,1],h);
    omega = acos(n(1) / norm(n)); % omega
    if(n(2) < 0)
        omega = 2*pi - omega;
    end
    
    w = acos(dot(n,ecc_vec) / (norm(n) * e)); % w
    if(ecc_vec(3) < 0)
        w = 2*pi - w;
    end
    
    v = acos(dot(ecc_vec,r) / (norm(r) * e)); % v
    if(dot(r,r_dot) < 0)
        w = 2*pi - w;
    end
else
    omega = 0;
    w = 0;
    v = 0;
end

== matlab function OrbitSimV1_export/Atomic Subsystem3/Wheel inertias/V_s1 ==
  data: I_w input; V_s output; V_w input; I_s input
function V_s = fcn(I_w, V_w, I_s)
V_s = (I_w * V_w) / I_s;

== matlab function OrbitSimV1_export/Atomic Subsystem3/Wheel inertias/V_s2 ==
  data: I_w input; V_s output; V_w input; I_s input
function V_s = fcn(I_w, V_w, I_s)
V_s = (I_w * V_w) / I_s;

== matlab function OrbitSimV1_export/Atomic Subsystem3/magnitude1 ==
  data: v input; mag output
function mag = fcn(v)

mag = sqrt(v(1)^2+v(2)^2+v(3)^2);

== matlab function OrbitSimV1_export/Altitude ==
  data: x input; alt output; y input; z input
function alt = fcn(x, y, z)

alt = sqrt(x^2 + y^2 + z^2) - (6.3781*10^6);

== matlab function OrbitSimV1_export/Atomic Subsystem3/Atomic Subsystem1/e2axis ==
  data: heading input; pitch input; roll input; vector output

function vector = e2axis(heading, pitch, roll)

eul = [heading -pitch roll];
coder.extrinsic('eul2rotm');
coder.extrinsic('rotm2axang');
rotm = eul2rotm(eul,'ZYX');
v = rotm2axang(rotm);
vector = [0;0;0;0];
vector(1) = v(1);
vector(2) = v(2);
vector(3) = v(3);
vector(4) = v(4);

end

== matlab function OrbitSimV1_export/Atomic Subsystem3/Atomic Subsystem1/vector creator ==
  data: mag_vec input; vec output
function vec = fcn(mag_vec)

cos_theta = mag_vec(3) / sqrt(mag_vec(1)^2+mag_vec(2)^2+mag_vec(3)^2);
theta = acos(cos_theta);
vec = [-mag_vec(2); mag_vec(1); 0; theta];

== matlab function OrbitSimV1_export/Atomic Subsystem3/Atomic Subsystem2/expander ==
  data: u input; u_x output; u_y output; u_z output
function [u_x,u_y,u_z] = fcn(u)

u_x = u(1);
u_y = u(2);
u_z = u(3);

== matlab function OrbitSimV1_export/Atomic Subsystem3/Atomic Subsystem2/expander1 ==
  data: u input; u_x output; u_y output; u_z output
function [u_x,u_y,u_z] = fcn(u)

u_x = u(1);
u_y = u(2);
u_z = u(3);

== matlab function OrbitSimV1_export/Atomic Subsystem3/Atomic Subsystem2/expander2 ==
  data: u input; u_x output; u_y output; u_z output
function [u_x,u_y,u_z] = fcn(u)

u_x = u(1);
u_y = u(2);
u_z = u(3);
